simulink model "Subsystem"  (R2020b)
settings: Solver=FixedStepAuto  StartTime=0.0  StopTime=10.0  FixedStep=0.1  MaxStep=.001  RelTol=1e-3
settings Model: Creator=SAGAR  LastModifiedBy=SAGAR
settings DataIOCC: SaveOutput=off  SaveTime=off

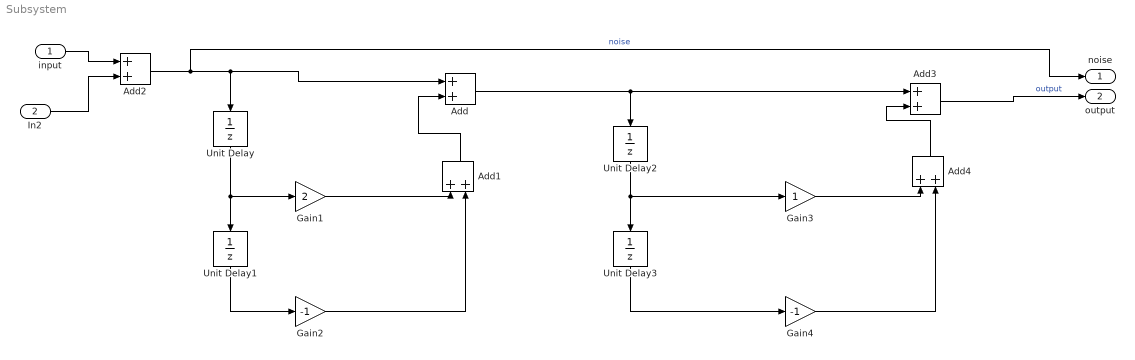
== system Subsystem ==
  input : Inport  OutDataTypeStr=double  PortDimensions=1  SampleTime=[0,1]
  In2 : Inport  Port=2  OutDataTypeStr=double  PortDimensions=1  SampleTime=[0.10000000000000001,0]
  Add{,1..4} (5 alike) : Sum
  Gain1 : Gain  Gain=2
  Gain2 : Gain  Gain=-1
  Gain3 : Gain
  Gain4 : Gain  Gain=-1
  Unit Delay{,1..3} (4 alike) : UnitDelay  SampleTime=-1  HasFrameUpgradeWarning=on
  noise : Outport  OutDataTypeStr=double  PortDimensions=1  SampleTime=[0.10000000000000001,0]
  output : Outport  Port=2  OutDataTypeStr=double  PortDimensions=1  SampleTime=[0.10000000000000001,0]
  wires:
  Gain4/1 -> Add4/2
  Add/1 -> Unit Delay2/1, Add3/1
  Unit Delay/1 -> Unit Delay1/1, Gain1/1
  Add1/1 -> Add/2
  Add2/1 -> Unit Delay/1, Add/1, noise/1  "noise"
  Gain3/1 -> Add4/1
  Unit Delay2/1 -> Unit Delay3/1, Gain3/1
  Gain1/1 -> Add1/1
  Unit Delay1/1 -> Gain2/1
  Gain2/1 -> Add1/2
  Add4/1 -> Add3/2
  input/1 -> Add2/1
  Unit Delay3/1 -> Gain4/1
  Add3/1 -> output/1  "output"
  In2/1 -> Add2/2
